simulink model "BackStepping_ex1_2_DesignComparison"  (R2021a)
settings: Solver=VariableStepAuto  StartTime=0.0  StopTime=30  RelTol=1e-3
settings Model: Creator=JianFongLee  LastModifiedBy=JianFongLee

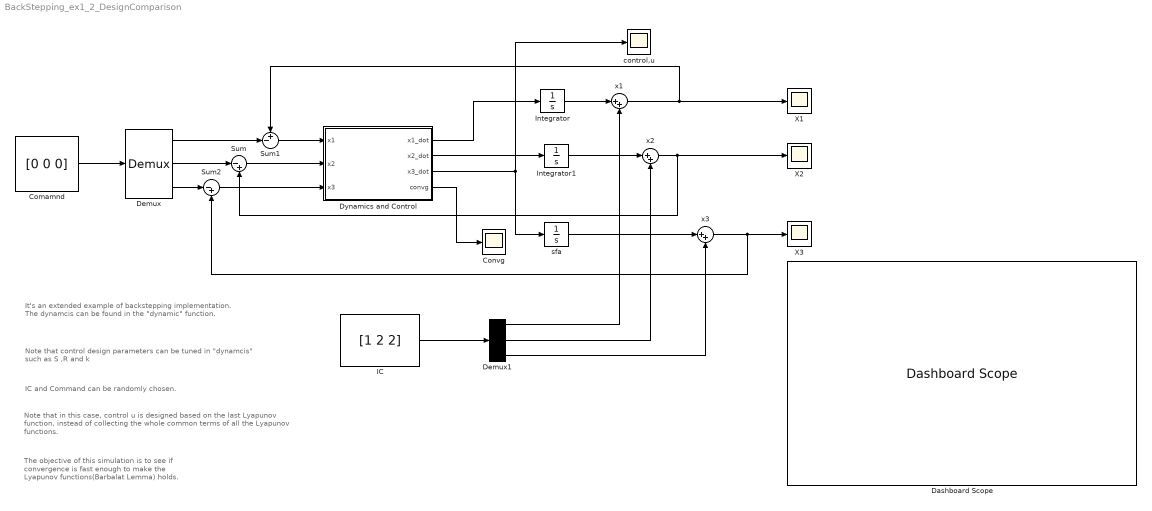
== system BackStepping_ex1_2_DesignComparison ==
  note: IC and Command can be randomly chosen.
  note: Note that control design parameters can be tuned in "dynamcis"
      | such as S ,R and k
  note: It's an extended example of backstepping implementation.
      | The dynamcis can be found in the "dynamic" function.
  note: The objective of this simulation is to see
      | if convergence is fast enough to make the
      | Lyapunov functions(Barbalat Lemma) holds.
  note: Note that in this case, control u is designed based on the
      |  last Lyapunov function, instead of collecting the whole common terms
      | of all the Lyapunov functions.
  Comamnd : Constant  Value=[0 0 0]
  Convg : Scope
  Dashboard Scope : DashboardScope
  Demux : Demux  Outputs=3
      settings: DisplayOption=none
  Demux1 : Demux  Outputs=3
      settings: DisplayOption=none
  Dynamics and Control : MATLAB Function  TreatAsAtomicUnit=on
  IC : Constant  Value=[1 2 2]
  Integrator : Integrator
  Integrator1 : Integrator
  Sum : Sum  Inputs=|-+
  Sum1 : Sum  Inputs=+-|
  Sum2 : Sum  Inputs=|-+
  X1 : Scope
  X2 : Scope
  X3 : Scope
  control,u : Scope
  sfa : Integrator
  x1 : Sum  Inputs=|++
  x2 : Sum  Inputs=|++
  x3 : Sum  Inputs=|++
  wires:
  Dynamics and Control/1(x1_dot) -> Integrator/1
  Dynamics and Control/2(x2_dot) -> Integrator1/1
  Sum/1 -> Dynamics and Control/2(x2)
  Sum1/1 -> Dynamics and Control/1(x1)
  IC/1 -> Demux1/1
  Demux1/1 -> x1/2
  Integrator/1 -> x1/1
  x1/1 -> X1/1, Sum1/1
  Integrator1/1 -> x2/1
  x2/1 -> Sum/2, X2/1
  Demux1/2 -> x2/2
  Comamnd/1 -> Demux/1
  Demux/1 -> Sum1/2
  Demux/2 -> Sum/1
  Demux/3 -> Sum2/1
  Sum2/1 -> Dynamics and Control/3(x3)
  x3/1 -> X3/1, Sum2/2
  Dynamics and Control/3(x3_dot) -> sfa/1, control,u/1
  sfa/1 -> x3/1
  Demux1/3 -> x3/2
  Dynamics and Control/4(convg) -> Convg/1

== matlab function BackStepping_ex1_2_DesignComparison/Dynamics and Control ==
  data: x1 input; x1_dot output; x2 input; x2_dot output; x3 input; x3_dot output; convg output
function [x1_dot,x2_dot, x3_dot, convg]= dynamics(x1, x2, x3)
x1_Dum= x1^2 - x1^3 + x2;  %%% Dunmmy for the Dynamics of x1_dot

%%% Parameters determination
k = 3; %%% Choose k > 0 
S = 1;   %%% S == 1 is the sweetspot
R = 10;  %% Maximum output of u

%%% Control u here(Two u represent 2 different designs)
P = x1 + 2*x1^3 - 2*x1^4 + 2*x1*x2;
P_dot = x1_Dum * (1 + 6*x1^2 - 8*x1^3 + 2*x2) + 2*x1*x3;
u = -1*P_dot - x2 - x1^2 - k*(x3+P)^S;  %%% Design for assuring convergence
%u = -1*P_dot - k*(x3+P)^S;         %%% Design by presumming convergence
%%% The lower 'u' is a bad design becasue it only assures convergence of x3
%%% It ignores the convergence of x2, so it creates oscillation

%%% Add a control output restriction
if abs(u) > abs(R)
   if u>0
       u = abs(R);
   else
       u = -1*abs(R);
   end
end

%%% Compute dynamics
x1_dot = x1_Dum;              %%% Dynamics of x1_dot
x2_dot = x3;                %%% Dynamics of x2_dot
x3_dot = u;                 %%% Dynamics of x3_dot
convg = abs(x3+P) + abs(x1+x2^2);   %%%Show if convergences hold

%%% Lynapunov functions
%%% V =     V     +        V1      +       V2
%%%   =  0.5*x1^2 + 0.5*(x1+x2^2)^2 + 0.5*(x3+P)^2;

%%% Note that u = -1*P_dot - x2 - x1^2 - k*(x3+P)^S;
%%% is designed on collective terms,
%%% which to assure V0_dot,V1_dot would be g.n.d 

%%% Note that u = -1*P_dot - k*(x3+P)^S;
%%% is designed soly on V3 in this case,
%%% which presumes x2 would be converged, however it's not. 

%%% Notation on S, the power determines how radical V_dot is
%%% S therotically could be any odd greater than 0,
%%% but experiments show that S = 3 or 5 would lead to significant oscillation
